simulink model "sampleModel346"  (R2021b)
settings: Solver=VariableStepAuto  StartTime=0.0  StopTime=10.0  RelTol=1e-3
undefined symbols (not defined in the file or in its folder): DiscIntNeverNeededParam, Newton, Raphson
libraries: simulink x5
settings Model: Creator=user  LastModifiedBy=user

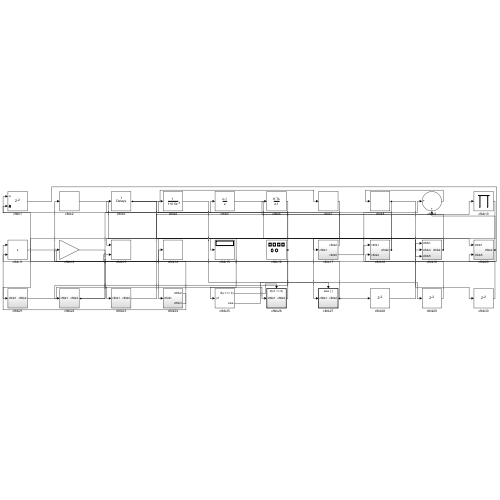
[thumbnail: Simulink's stored preview of the top-level diagram]
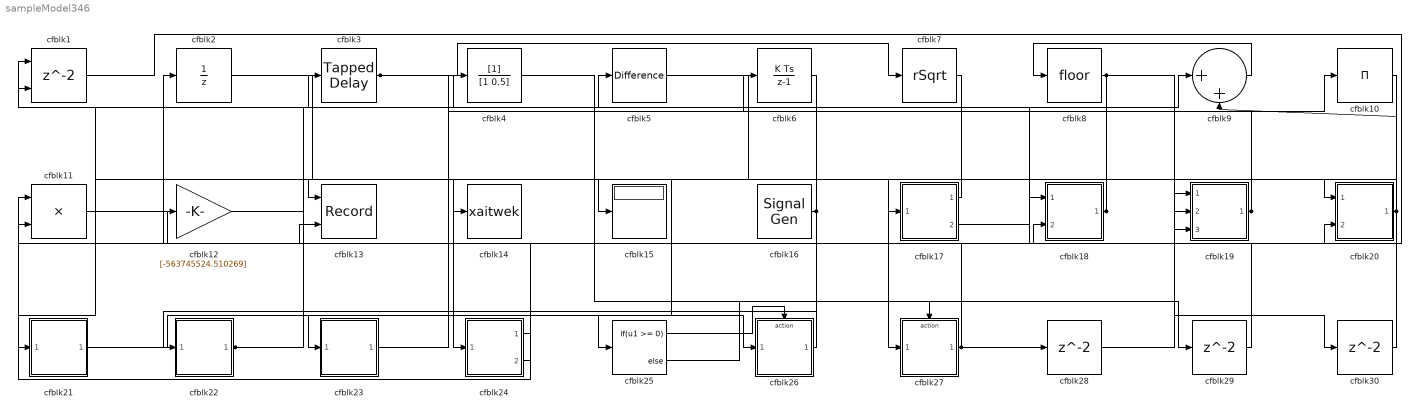
== system sampleModel346 ==
  cfblk1 : Delay  ShowEnablePort=on  SampleTime=1
      settings: InputPortMap=u0,e6
  cfblk10 : Product  Inputs=*
  cfblk11 : Product  Inputs=**
  cfblk12 : Gain  Gain=[-563745524.510269]
  cfblk13 : Record  FileSettingsInternal="{\"entries\":[{\"content\":{\"excelSettings\":{\"content\":{},\"type\":\"Streamout.ExcelSettings\"}},\"type\":\"Streamout.FileSettingStorage\",\"uuid\":\"2113a4ae-a6fb-4ee9-81b0-3c11124e163c\"}],\"packageUris\":[\"http://schema.mathworks.com/mf0/streamout_blocks/R2020a\"],\"version\":\"1.0\"}"  Layout=[1 1]  SignalsInternal="{\"entries\":[{\"content\":{\"signals\":[{\"content\":{\"blockPath\":[\"sampleModel346/cfblk13\"],\"channel\":[],\"dimensions\":[1],\"domain\":\"sampleModel346/cfblk13\",\"lineColor\":\"#a2142f\",\"plots\":[1],\"port\":1,\"sid\":[\"\"],\"signalID\":14497,\"signalName\":\"cfblk18\"},\"type\":\"RecordBlkView.Signal\",\"uuid\":\"35f50a97-31e6-440d-8ef6-b82915ee1f38\"},{\"content\":{\"blockPath\":[\"sampleModel346/cfblk13\"],\"channel\":[],\"dimensions\":[1],\"domain\":\"sampleModel346/cfblk13\",\"lineColor\":\"#139fff\",\"plots\":[1],\"port\":2,\"sid\":[\"\"],\"signalID\":14501,\"signalName\":\"cfblk11\"},\"type\":\"RecordBlkView.Signal\",\"uuid\":\"a5d959cf-dd60-4373-856b-49f2df5a3ca0\"}]},\"type\":\"RecordBlkView.InputSignals\",\"uuid\":\"576ef5b6-f15b-47c0-abe2-34e59efa76ff\"}],\"packageUris\":[\"http://schema.mathworks.com/mf0/streamout_blocks/R2020a\"],\"version\":\"1.0\"}"  VisualizationBindings="{\"xyplotplugin\":{\"info\":[{\"series\":[{\"bindingParametersList\":[{\"parameter\":\"X-Axis\",\"signalID\":14497,\"signalName\":\"cfblk18\"},{\"parameter\":\"Y-Axis\",\"signalID\":14501,\"signalName\":\"cfblk11\"}],\"seriesID\":12264}],\"subplotID\":1}]}}"  CompatibilityTag=XY
  cfblk14 : ToWorkspace  VariableName=xaitwek  SaveFormat=Timeseries  SampleTime=-1
  cfblk15 : Display
  cfblk16 : SignalGenerator  WaveForm=sawtooth  Amplitude=[-641970928.023362]
  cfblk17 : Subsystem
  cfblk18 : Subsystem
  cfblk19 : Subsystem
  cfblk2 : UnitDelay  HasFrameUpgradeWarning=on
  cfblk20 : Subsystem
  cfblk21 : Subsystem
  cfblk22 : Subsystem
  cfblk23 : Subsystem
  cfblk24 : Subsystem
  cfblk25 : If  IfExpression=u1 >= 0  SampleTime=1
  cfblk26 : Subsystem  TreatAsAtomicUnit=on
  cfblk27 : Subsystem  TreatAsAtomicUnit=on
  cfblk28 : Delay  SampleTime=1
  cfblk29 : Delay  SampleTime=1
  cfblk3 : simulink/Discrete/Tapped Delay  vinit=0.0  samptime=-1  NumDelays=1  DelayOrder=Oldest  includeCurrent=off
  cfblk30 : Delay  SampleTime=1
  cfblk4 : DiscreteFilter  SampleTime=1
  cfblk5 : simulink/Discrete/Difference  ICPrevInput=0.0  OutMin=[]  OutMax=[]  OutDataTypeStr=Inherit: Inherit via back propagation  OutDataType=fixdt(1, 16)  OutScaling=2^-10  DoSatur=off
  cfblk6 : DiscreteIntegrator  ICPrevOutput=DiscIntNeverNeededParam  ICPrevScaledInput=DiscIntNeverNeededParam
  cfblk7 : Sqrt  Operator=rSqrt  AlgorithmType=Newton-Raphson  SaturateOnIntegerOverflow=on
  cfblk8 : Rounding
  cfblk9 : Sum  Inputs=|++
  wires:
  cfblk21/1(cfblk2) -> cfblk23/1(cfblk1)
  cfblk10/1 -> cfblk24/1(cfblk1)
  cfblk22/1(cfblk2) -> cfblk14/1, cfblk5/1
  cfblk2/1 -> cfblk15/1
  cfblk18/1(cfblk2) -> cfblk13/1, cfblk3/1
  cfblk5/1 -> cfblk20/1(cfblk1)
  cfblk19/1(cfblk2) -> cfblk6/1, cfblk17/1(cfblk1)
  cfblk8/1 -> cfblk27/1(cfblk1), cfblk30/1
  cfblk11/1 -> cfblk13/2
  cfblk3/1 -> cfblk7/1, cfblk19/2(cfblk4), cfblk19/3(cfblk5)
  cfblk12/1 -> cfblk26/1(cfblk1)
  cfblk6/1 -> cfblk25/1
  cfblk27/1(cfblk2) -> cfblk11/2, cfblk28/1
  cfblk26/1(cfblk2) -> cfblk2/1
  cfblk24/1(cfblk2) -> cfblk11/1
  cfblk1/1 -> cfblk20/2(cfblk5)
  cfblk7/1 -> cfblk21/1(cfblk1)
  cfblk24/2(cfblk3) -> cfblk12/1
  cfblk17/1(cfblk2) -> cfblk4/1
  cfblk9/1 -> cfblk8/1
  cfblk16/1 -> cfblk22/1(cfblk1), cfblk1/1
  cfblk20/1(cfblk2) -> cfblk18/2(cfblk4), cfblk9/2
  cfblk17/2(cfblk5) -> cfblk9/1
  cfblk23/1(cfblk2) -> cfblk10/1
  cfblk25/1 -> cfblk26/Action
  cfblk25/2 -> cfblk27/Action
  cfblk28/1 -> cfblk19/1(cfblk1)
  cfblk4/1 -> cfblk29/1
  cfblk29/1 -> cfblk18/1(cfblk1)
  cfblk30/1 -> cfblk1/2

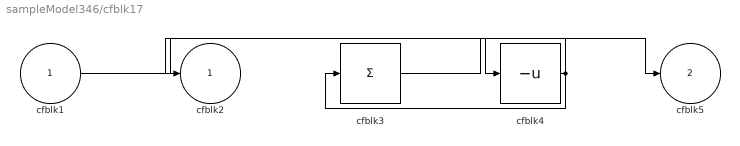
== system sampleModel346/cfblk17 ==
  cfblk1 : Inport
  cfblk3 : Sum  Inputs=+
  cfblk4 : UnaryMinus
  cfblk2 : Outport
  cfblk5 : Outport  Port=2
  wires:
  cfblk1/1 -> cfblk4/1
  cfblk4/1 -> cfblk3/1, cfblk2/1
  cfblk3/1 -> cfblk5/1

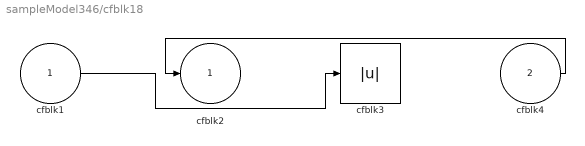
== system sampleModel346/cfblk18 ==
  cfblk1 : Inport
  cfblk4 : Inport  Port=2
  cfblk3 : Abs
  cfblk2 : Outport
  wires:
  cfblk4/1 -> cfblk2/1
  cfblk1/1 -> cfblk3/1

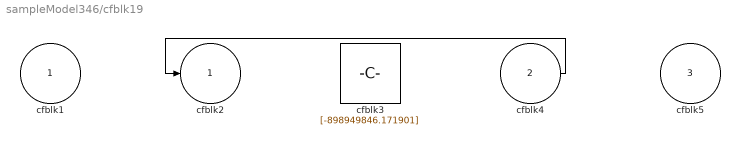
== system sampleModel346/cfblk19 ==
  cfblk1 : Inport
  cfblk4 : Inport  Port=2
  cfblk5 : Inport  Port=3
  cfblk3 : Constant  Value=[-898949846.171901]  SampleTime=1
  cfblk2 : Outport
  wires:
  cfblk4/1 -> cfblk2/1

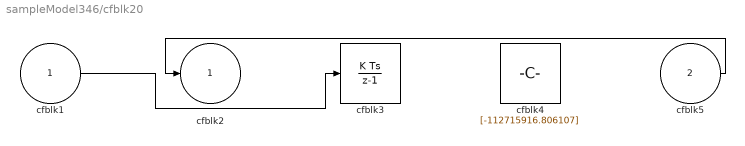
== system sampleModel346/cfblk20 ==
  cfblk1 : Inport
  cfblk5 : Inport  Port=2
  cfblk3 : DiscreteIntegrator  ICPrevOutput=DiscIntNeverNeededParam  ICPrevScaledInput=DiscIntNeverNeededParam
  cfblk4 : Constant  Value=[-112715916.806107]  SampleTime=1
  cfblk2 : Outport
  wires:
  cfblk5/1 -> cfblk2/1
  cfblk1/1 -> cfblk3/1

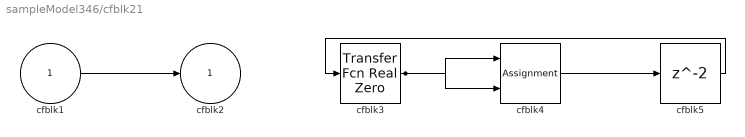
== system sampleModel346/cfblk21 ==
  cfblk1 : Inport
  cfblk3 : simulink/Discrete/Transfer Fcn Real Zero  ZeroZ=0.75  ICPrevInput=0.0  DoSatur=off
      settings: SourceProductBaseCode=SL
  cfblk4 : Assignment  DiagnosticForDimensions=Warning  IndexOptions=Index vector (dialog)  Indices=1  OutputSizes=1
  cfblk5 : Delay  SampleTime=1
  cfblk2 : Outport
  wires:
  cfblk1/1 -> cfblk2/1
  cfblk3/1 -> cfblk4/1, cfblk4/2
  cfblk4/1 -> cfblk5/1
  cfblk5/1 -> cfblk3/1

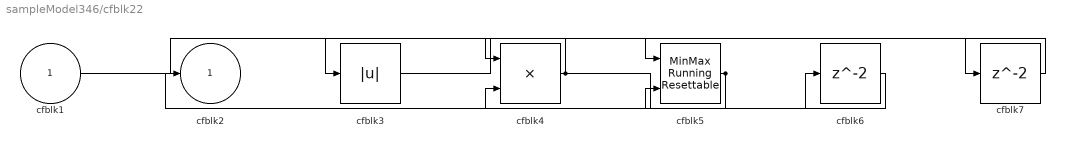
== system sampleModel346/cfblk22 ==
  cfblk1 : Inport
  cfblk3 : Abs
  cfblk4 : Product  Inputs=**
  cfblk5 : simulink/Math Operations/MinMax Running Resettable  Function=min  vinit=0.0
  cfblk6 : Delay  SampleTime=1
  cfblk7 : Delay  SampleTime=1
  cfblk2 : Outport
  wires:
  cfblk1/1 -> cfblk5/1
  cfblk5/1 -> cfblk2/1, cfblk4/2
  cfblk4/1 -> cfblk3/1, cfblk6/1
  cfblk6/1 -> cfblk5/2
  cfblk3/1 -> cfblk7/1
  cfblk7/1 -> cfblk4/1

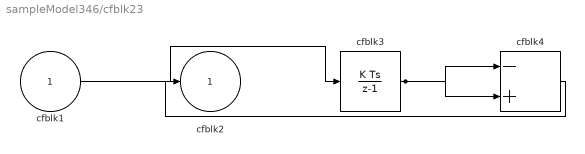
== system sampleModel346/cfblk23 ==
  cfblk1 : Inport
  cfblk3 : DiscreteIntegrator  ICPrevOutput=DiscIntNeverNeededParam  ICPrevScaledInput=DiscIntNeverNeededParam
  cfblk4 : Sum  Inputs=-+
  cfblk2 : Outport
  wires:
  cfblk1/1 -> cfblk3/1
  cfblk4/1 -> cfblk2/1
  cfblk3/1 -> cfblk4/1, cfblk4/2

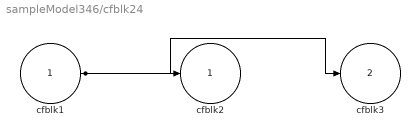
== system sampleModel346/cfblk24 ==
  cfblk1 : Inport
  cfblk2 : Outport
  cfblk3 : Outport  Port=2
  wires:
  cfblk1/1 -> cfblk3/1, cfblk2/1

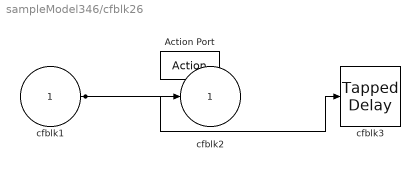
== system sampleModel346/cfblk26 ==
  cfblk1 : Inport
  Action Port : ActionPort  ActionPortLabel=if(u1 >= 0)
  cfblk3 : simulink/Discrete/Tapped Delay  vinit=0.0  samptime=-1  NumDelays=1  DelayOrder=Oldest  includeCurrent=off
  cfblk2 : Outport
  wires:
  cfblk1/1 -> cfblk2/1, cfblk3/1

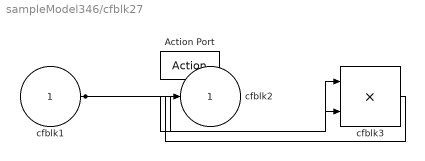
== system sampleModel346/cfblk27 ==
  cfblk1 : Inport
  Action Port : ActionPort  ActionPortLabel=else
  cfblk3 : Product  Inputs=**
  cfblk2 : Outport
  wires:
  cfblk1/1 -> cfblk3/1, cfblk3/2
  cfblk3/1 -> cfblk2/1
